simulink model "MultiRobotSwarmSimulink"  (R2025b)
settings: Solver=ode45  StartTime=0.0  StopTime=60  FixedStep=0.05  RelTol=1e-3
settings Model: Creator=chandansheikder  LastModifiedBy=chandansheikder

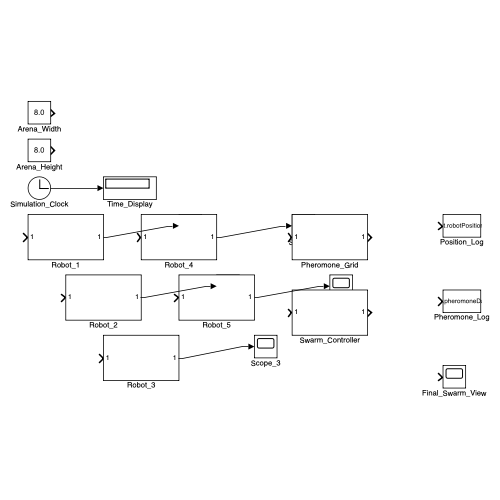
[thumbnail: Simulink's stored preview of the top-level diagram]
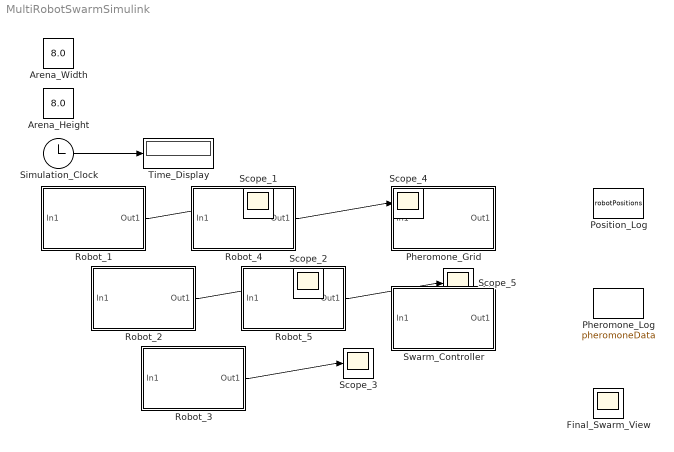
== system MultiRobotSwarmSimulink ==
  Arena_Height : Constant  Value=8.0
  Arena_Width : Constant  Value=8.0
  Final_Swarm_View : Scope
  Pheromone_Grid : Subsystem
  Pheromone_Log : ToWorkspace  VariableName=pheromoneData  SaveFormat=Timeseries  SampleTime=-1
  Position_Log : ToWorkspace  VariableName=robotPositions  SaveFormat=Timeseries  SampleTime=-1
  Robot_1 : Subsystem
  Robot_2 : Subsystem
  Robot_3 : Subsystem
  Robot_4 : Subsystem
  Robot_5 : Subsystem
  Scope_{1..5} (5 alike) : Scope
  Simulation_Clock : Clock
  Swarm_Controller : Subsystem
  Time_Display : Display
  wires:
  Simulation_Clock/1 -> Time_Display/1
  Robot_1/1(Out1) -> Scope_1/1
  Robot_2/1(Out1) -> Scope_2/1
  Robot_3/1(Out1) -> Scope_3/1
  Robot_4/1(Out1) -> Scope_4/1
  Robot_5/1(Out1) -> Scope_5/1

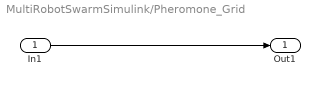
== system MultiRobotSwarmSimulink/Pheromone_Grid ==
  In1 : Inport
  Out1 : Outport
  wires:
  In1/1 -> Out1/1

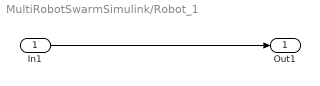
== system MultiRobotSwarmSimulink/Robot_1 ==
  In1 : Inport
  Out1 : Outport
  wires:
  In1/1 -> Out1/1

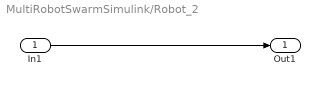
== system MultiRobotSwarmSimulink/Robot_2 ==
  In1 : Inport
  Out1 : Outport
  wires:
  In1/1 -> Out1/1

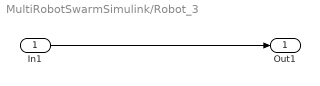
== system MultiRobotSwarmSimulink/Robot_3 ==
  In1 : Inport
  Out1 : Outport
  wires:
  In1/1 -> Out1/1

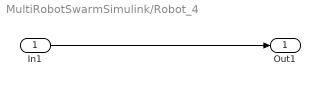
== system MultiRobotSwarmSimulink/Robot_4 ==
  In1 : Inport
  Out1 : Outport
  wires:
  In1/1 -> Out1/1

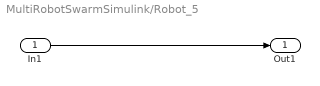
== system MultiRobotSwarmSimulink/Robot_5 ==
  In1 : Inport
  Out1 : Outport
  wires:
  In1/1 -> Out1/1

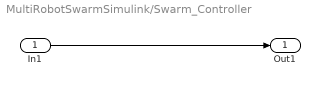
== system MultiRobotSwarmSimulink/Swarm_Controller ==
  In1 : Inport
  Out1 : Outport
  wires:
  In1/1 -> Out1/1
